simulink model "UUVModel"  (R2024b)
settings: Solver=ode4  StartTime=0.0  StopTime=100  FixedStep=0.001  RelTol=1e-3
PreLoadFcn:
  | [filepath,name,ext]  = fileparts(get_param(bdroot, 'FileName'));
  | InitFileName=[name,'_init.m'];
  | cd(filepath);
InitFcn:
  | [filepath,name,ext]  = fileparts(get_param(bdroot, 'FileName'));
  | InitFileName=[name,'_init.m'];
  | cd(filepath);
  | try
  | run(InitFileName);
  | end
values from neighbouring files (symbols this model uses):
  ESC = [ESC,ESCTmp]    [UUVModel_init.m]
  ModelParam_envAltitude = -600    [UUVModel_init.m]
  ModelParam_GPSLatLong = [ModelParam_envLatitude ModelParam_envLongitude]    [UUVModel_init.m]
  ModelParam_uavJ = [ModelParam_uavJxx,0,0;0,ModelParam_uavJyy,0;0,0,ModelParam_uavJzz]    [UUVModel_init.m]
  ModelParam_uavMass = 11.0    (= 11)    [UUVModel_init.m]
  ModelParam_uavType = int16(600)    [UUVModel_init.m]
  motor = [motor,motorTmp]    [UUVModel_init.m]
undefined symbols (not defined in the file or in its folder): Earth, ModelParam_timeSamp, UUV, WGS84
libraries: RflySimModelLab x15, aerolibtransform2 x2, aerolibatmos2 x2, sharedtransform x1, shared6dof x1, aerolibconvert2 x1, aerolibobsolete x1, aerolibasang x1, aerolibnav x1, aerolibgravity2 x1
(part 1 of 2)
settings Model: Creator=Jinrui  LastModifiedBy=12043
settings SolverCC: AlgebraicLoopSolver=TrustRegion
settings DataIOCC: ReturnWorkspaceOutputs=off
settings OptimizationCC: ReuseModelBlockBuffer=off  ZeroExternalMemoryAtStartup=off  ZeroInternalMemoryAtStartup=off  EfficientTunableParamExpr=on
settings DebuggingCC: ParameterTunabilityLossMsg=error  UnconnectedInputMsg=warning  UnconnectedOutputMsg=warning  UnconnectedLineMsg=warning  ArithmeticOperatorsInVariantConditions=warning
settings ModelReferenceCC: EnableRefExpFcnMdlSchedulingChecks=on
settings SFSimCC: SimUseLocalCustomCode=off  MATLABDynamicMemAlloc=off  CustomCodeUndefinedFunction=UseInterfaceOnly  SimTargetLang=C++
settings RTWCC: Description=Embedded Coder  SystemTargetFile=ert.tlc  GenerateMakefile=off  PackageGeneratedCodeAndArtifacts=on  PackageName=MulticopterModel  TemplateMakefile=ert_default_tmf  RTWUseLocalCustomCode=off  TargetLang=C++  RTWCompilerOptimization=on  GPUComputeCapability=3.5
settings CodeAppCC: ForceParamTrailComments=on  OperatorAnnotations=on  SimulinkDataObjDesc=on  SFDataObjDesc=on  MATLABFcnDesc=on  InsertBlockDesc=on  StateflowObjectComments=on  MATLABSourceComments=on
settings ERTTargetCC: TargetLangStandard=C++03 (ISO)  MultiwordLength=2048  GenerateSampleERTMain=on  CodeInterfacePackaging=C++ class  SupportContinuousTime=on  InlinedParameterPlacement=Hierarchical  MultiInstanceErrorCode=None  RootIOFormat=Structure reference  ERTCustomFileTemplate=example_file_process.tlc  ERTFilePackagingFormat=Compact  DynamicArrayContainerType=coder::array
settings SimscapeCC: SimscapeNormalizeSystem=off

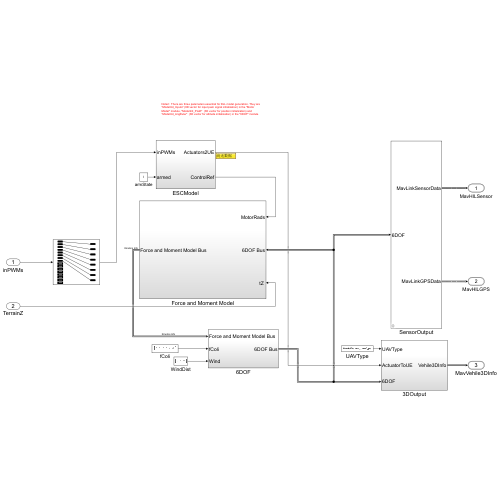
[thumbnail: Simulink's stored preview of the top-level diagram]
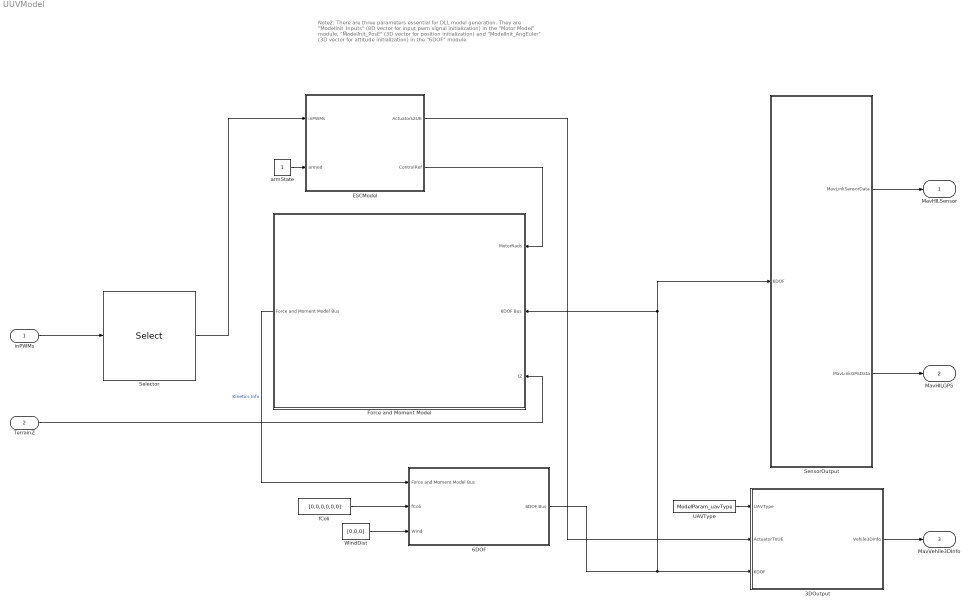
== system UUVModel ==
  note: Note2: There are three parameters essential for DLL model generation. They are "ModelInit_Inputs" (8D vector for input pwm signal initialization) in the "Motor Model" module, "ModelInit_PosE" (3D vector for position initialization) and "ModelInit_AngEuler" (3D vector for attitude initialization) in the "6DOF" module
  inPWMs : Inport  PortDimensions=16
  TerrainZ : Inport  Port=2
  3DOutput : Subsystem
  6DOF : Subsystem
  ESCModel : Subsystem
  Force and Moment Model : Subsystem
  Selector : Selector  InputPortWidth=16  IndexOptions=Index vector (dialog)  Indices=[1:8]  OutputSizes=1
  SensorOutput : Subsystem  mask{ModelParam_GPSLatLong=ModelParam_GPSLatLong, ModelParam_envAltitude=ModelParam_envAltitude}
      mask prompts: ModelParam_GPSLatLong "Initial latitude and longitude [deg]:"; ModelParam_envAltitude "Initial altitude [m]:"
      mask init:
      | ModelParam_GlobalNoiseGainSwitch =0.4;
      | %SimParam.timeACC=1;
      | %SimParam.timeStep=0.0001;
      | % SimParam.sonarSamp=0.1;
      | % SimParam.AngEularSamp=0.004;
      | % SimParam.AngRateSamp=0.004;
      | % SimParam.AccSensSamp=0.004;
      | % SimParam.GyroSensSamp=0.004;
      | % SimParam.AngQuaternSamp=0.004;
      | % SimParam.BaroSamp=0.008;
      | % SimParam.AngEulerSamp=0.004;
      | ModelParam_timeSampBaro = 0.01;
      | ModelParam_timeSampTurbWind = 0.01;
      | ModelParam_BusSampleRate = 0.001;
      | 
      | 
      | 
      | %%%ModelParam_BattModelEnable=int8(0);
      | %ModelParam_BattAuxCurrent=0.5;
      | %ModelParam_BattCells=3;
      | %ModelParam_BattCapacity=0.55;   %%这一项从模型配置界面传输给定
      | ModelParam_BattHoverMinutes=18;
      | ModelParam_BattHoverThr=0.609;
      | 
      | %GPS Parameter
      | ModelParam_GPSEphFinal=0.3;
      | ModelParam_GPSEpvFinal=0.4;
      | ModelParam_GPSFix3DFix=3;
      | ModelParam_GPSSatsVisible=10;
      | 
      | 
      | %Noise Parameter
      | ModelParam_noisePowerAccel = [0.001,0.001,0.003];%顺序 xyz 下同  不要修改这里
      | ModelParam_noiseSampleTimeAccel = 0.001;
      | %ModelParam_noiseLowPassFilterCoeAccel = 0.0001;
      | ModelParam_noisePowerOffGainAccel = 0.04;
      | ModelParam_noisePowerOffGainAccelZ = 0.03;
      | ModelParam_noisePowerOnGainAccel = 0.8;
      | ModelParam_noisePowerOnGainAccelZ = 4.5;
      | 
      | 
      | ModelParam_noisePowerGyro = [0.00001,0.00001,0.00001];%不要修改这里
      | ModelParam_noiseSampleTimeGyro = 0.001;
      | %ModelParam_noiseLowPassFilterCoeGyro = 0.0001;
      | ModelParam_noisePowerOffGainGyro = 0.02;
      | ModelParam_noisePowerOffGainGyroZ = 0.025;
      | ModelParam_noisePowerOnGainGyro = 2;%3.2;
      | ModelParam_noisePowerOnGainGyroZ = 1;
      | 
      | 
      | 
      | ModelParam_noisePowerMag = [0.00001,0.00001,0.00001];%不要修改这里
      | ModelParam_noiseSampleTimeMag = 0.01;
      | %ModelParam_noiseLowPassFilterCoeMag = 0.02;%暂时没有使用
      | ModelParam_noisePowerOffGainMag = 0.02;
      | ModelParam_noisePowerOffGainMagZ = 0.035;
      | ModelParam_noisePowerOnGainMag = 0.025;
      | ModelParam_noisePowerOnGainMagZ = 0.05;
      | 
      | 
      | 
      | ModelParam_noisePowerIMU=0;%IMU噪声，这里是白噪声，这里是经过归一化
      | 
      | ModelParam_noiseUpperGPS=0.5;  %GPS定位误差噪声，均匀噪声，这里填x,y,z的波动上限，单位是m
      | ModelParam_noiseGPSSampTime=0.02;%默认0.05
      | 
      | ModelParam_noiseUpperBaro=0; %气压计噪声，均匀噪声，这里填高度的波动上限，单位是m
      | ModelParam_noiseBaroSampTime=0.02;%气压计噪声更新频率，，默认0.05
      | ModelParam_noiseBaroCoupleWithSpeed=0;%气压计测量高度与动压关系，也就是风速与气压计掉高模型的系数，当前参数0.008飞机10m/s掉高1m
      | 
      | ModelParam_noiseUpperWindBodyRatio=0;%风波动系数，风速*(1+该系数)
      | ModelParam_noiseWindSampTime=0.001;
      | 
      | %%ModelParam_envGravityAcc = 9.81;
      | ModelParam_envAirDensity = 1.225;    %还没有用到
      | ModelParam_envDiffPressure = 0; % Differential pressure (airspeed) in millibar
      | ModelParam_noiseTs = 0.001;
      | 
      | %ModelParam_FailModelStartT = 5;
      | %ModelParam_FailModelLastT = 5;
  UAVType : Constant  Value=ModelParam_uavType
  WindDist : Constant  Value=[0,0,0]
  armState : Constant
  fColi : Constant  Value=[0,0,0,0,0,0]
  MavHILSensor : Outport  OutDataTypeStr=Bus: MavLinkSensor  VectorParamsAs1DForOutWhenUnconnected=off
  MavHILGPS : Outport  Port=2  OutDataTypeStr=Bus: MavLinkGPS  VectorParamsAs1DForOutWhenUnconnected=off
  MavVehile3DInfo : Outport  Port=3  OutDataTypeStr=Bus: MavVehileInfo  VectorParamsAs1DForOutWhenUnconnected=off
  wires:
  SensorOutput/1(MavLinkSensorData) -> MavHILSensor/1
  3DOutput/1(Vehile3DInfo) -> MavVehile3DInfo/1
  SensorOutput/2(MavLinkGPSData) -> MavHILGPS/1
  ESCModel/2(ControlRef) -> Force and Moment Model/1(MotorRads)
  Force and Moment Model/1(Force and Moment Model Bus) -> 6DOF/1(Force and Moment Model Bus)  "Kinetics Info"
  armState/1 -> ESCModel/2(armed)
  TerrainZ/1 -> Force and Moment Model/3("tZ ")
  inPWMs/1 -> Selector/1
  Selector/1 -> ESCModel/1(inPWMs)
  UAVType/1 -> 3DOutput/1(UAVType)
  6DOF/1(6DOF Bus) -> 3DOutput/3(6DOF), SensorOutput/1(6DOF), Force and Moment Model/2(6DOF Bus)
  ESCModel/1(Actuators2UE) -> 3DOutput/2(ActuatorToUE)
  WindDist/1 -> 6DOF/3(Wind)
  fColi/1 -> 6DOF/2(fColi)

== system UUVModel/3DOutput ==
  UAVType : Inport
  ActuatorToUE : Inport  Port=2
  6DOF : Inport  Port=3
  Bus Selector : BusSelector  OutputSignals=Ve,Xe,Eular(rad),DCM,wb,dwb/dt,AccB,WindB
  Clock1 : Clock
  Terminator : Terminator
  Terminator1 : Terminator
  Vehile3DModel : Subsystem
  Vehile3DInfo : Outport  VectorParamsAs1DForOutWhenUnconnected=off
  wires:
  Bus Selector/4 -> Vehile3DModel/9(<DCM>)  "<DCM>"
  Bus Selector/5 -> Vehile3DModel/6(<wb>)  "<wb>"
  Bus Selector/2 -> Vehile3DModel/7(<Xe>)  "<Xe>"
  UAVType/1 -> Vehile3DModel/1(vehicleType)
  ActuatorToUE/1 -> Vehile3DModel/2(ActuatorToUE)
  Vehile3DModel/1(Vehile3DInfo) -> Vehile3DInfo/1
  Clock1/1 -> Vehile3DModel/3(runnedTime)
  Bus Selector/3 -> Vehile3DModel/4(<Eular(rad)>)  "<Eular(rad)>"
  Bus Selector/1 -> Vehile3DModel/8(<Ve>)  "<Ve>"
  Bus Selector/7 -> Vehile3DModel/5(<AccB>)  "<AccB>"
  6DOF/1 -> Bus Selector/1
  Bus Selector/6 -> Terminator/1  "<dwb/dt>"
  Bus Selector/8 -> Terminator1/1  "<WindB>"

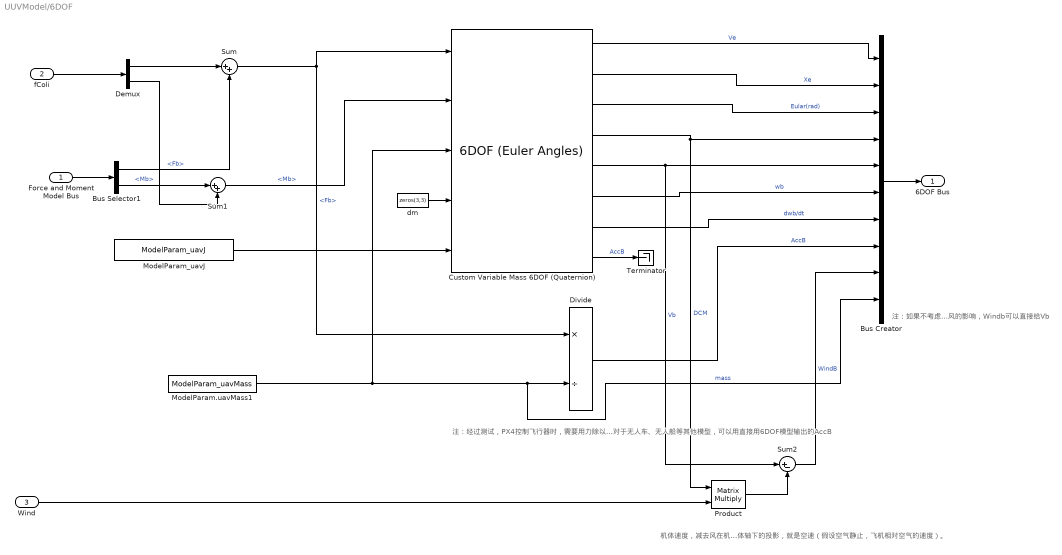
== system UUVModel/6DOF ==
  note: 注：如果不考虑风的影响，Windb可以直接给Vb
  note: 注：经过测试，PX4控制飞行器时，需要用力除以力矩的加速度去生成加速度计的数据，对于无人车、无人船等其他模型，可以用直接用6DOF模型输出的AccB
  note: 机体速度，减去风在机体轴下的投影，就是空速（假设空气静止，飞机相对空气的速度）。
  Force and Moment Model Bus : Inport
  fColi : Inport  Port=2
  Wind : Inport  Port=3
  Bus Creator : BusCreator  Inputs=10
  Bus Selector1 : BusSelector  OutputSignals=Fb,Mb
  Custom Variable Mass 6DOF (Quaternion) : shared6dof/6DOF (Euler Angles)  units=Metric (MKS)  mtype=Custom Variable  rep=Quaternion  xme_0=ModelInit_PosE  Vm_0=ModelInit_VelB  eul_0=ModelInit_AngEuler  pm_0=ModelInit_RateB  mass_0=ModelParam_uavMass  mass_e=0.5  mass_f=2.0  inertia=ModelParam_uavJ  inertia_e=eye(3)  inertia_f=2*eye(3)  k_quat=1.0  vre_flag=off  abi_flag=off  aMode=aMode  xme_statename=''  Vm_statename=''  eul_statename=''  quat_statename=''  pm_statename=''  mass_statename=''
  Demux : Demux  Outputs=2
  Divide : Product  Inputs=*/
  ModelParam.uavMass1 : Constant  Value=ModelParam_uavMass
  ModelParam_uavJ : Constant  Value=ModelParam_uavJ
  Product : Product  Multiplication=Matrix(*)
  Sum : Sum  Inputs=|++
  Sum1 : Sum  Inputs=|++
  Sum2 : Sum  Inputs=|+-
  Terminator : Terminator
  dm : Constant  Value=zeros(3,3)
  6DOF Bus : Outport  VectorParamsAs1DForOutWhenUnconnected=off
  wires:
  Bus Selector1/1 -> Sum/2  "<Fb>"
  Bus Selector1/2 -> Sum1/1  "<Mb>"
  Force and Moment Model Bus/1 -> Bus Selector1/1
  Demux/2 -> Sum1/2
  Demux/1 -> Sum/1
  fColi/1 -> Demux/1
  Custom Variable Mass 6DOF (Quaternion)/7 -> Bus Creator/7  "dwb/dt"
  Bus Creator/1 -> 6DOF Bus/1
  Custom Variable Mass 6DOF (Quaternion)/6 -> Bus Creator/6  "wb"
  Sum1/1 -> Custom Variable Mass 6DOF (Quaternion)/2  "<Mb>"
  Sum/1 -> Divide/1, Custom Variable Mass 6DOF (Quaternion)/1  "<Fb>"
  Custom Variable Mass 6DOF (Quaternion)/8 -> Terminator/1  "AccB"
  Custom Variable Mass 6DOF (Quaternion)/5 -> Sum2/1, Bus Creator/5  "Vb"
  Custom Variable Mass 6DOF (Quaternion)/4 -> Product/1, Bus Creator/4  "DCM"
  Custom Variable Mass 6DOF (Quaternion)/3 -> Bus Creator/3  "Eular(rad)"
  Custom Variable Mass 6DOF (Quaternion)/1 -> Bus Creator/1  "Ve"
  Custom Variable Mass 6DOF (Quaternion)/2 -> Bus Creator/2  "Xe"
  ModelParam.uavMass1/1 -> Bus Creator/10, Divide/2, Custom Variable Mass 6DOF (Quaternion)/3  "mass"
  Divide/1 -> Bus Creator/8  "AccB"
  Wind/1 -> Product/2
  Product/1 -> Sum2/2
  Sum2/1 -> Bus Creator/9  "WindB"
  dm/1 -> Custom Variable Mass 6DOF (Quaternion)/4
  ModelParam_uavJ/1 -> Custom Variable Mass 6DOF (Quaternion)/5

== system UUVModel/ESCModel ==
  note: 这个是输出给到UE用于舵机转动显示的，因此需要调整顺序到与UE对应，且修改单位到合适值。
  note: 输出的是8维向量
  inPWMs : Inport
  armed : Inport  Port=2
  ESC_All : Subsystem  AncestorBlock=RflySimModelLab/ESC_All  mask{ESCParam=ESC}
      mask prompts: ESCParam "电调参数"
      settings: LibrarySourceBlock=RflySimModelLab/ESC_All
  ToUEActuators : Subsystem
  Actuators2UE : Outport  VectorParamsAs1DForOutWhenUnconnected=off
  ControlRef : Outport  Port=2  VectorParamsAs1DForOutWhenUnconnected=off
  wires:
  inPWMs/1 -> ESC_All/1(inPWMs)
  ESC_All/1(MotorRads_reference) -> ToUEActuators/1(inMotorRads), ControlRef/1
  armed/1 -> ESC_All/2(armed)
  ToUEActuators/1(UERads) -> Actuators2UE/1

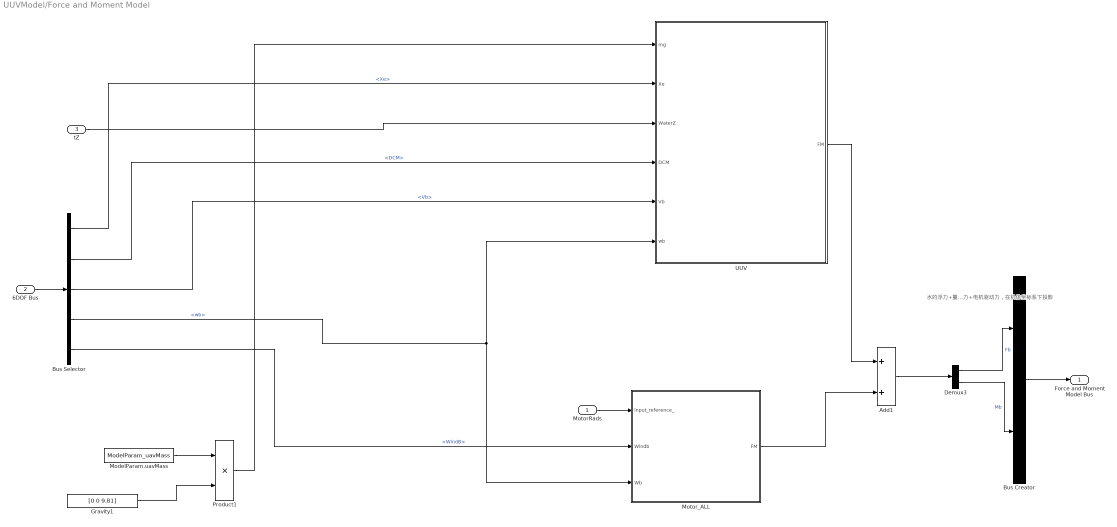
== system UUVModel/Force and Moment Model ==
  note: 水的浮力+重力+电机驱动力，在机体坐标系下投影
  MotorRads : Inport
  6DOF Bus : Inport  Port=2
  "tZ " : Inport  Port=3
  Add1 : Sum
  Bus Creator : BusCreator  Inputs=2
  Bus Selector : BusSelector  OutputSignals=Xe,DCM,Vb,wb,WindB
  Demux3 : Demux  Outputs=2
  Gravity1 : Constant  Value=[0 0 9.81]
  ModelParam.uavMass : Constant  Value=ModelParam_uavMass
  Motor_ALL : Subsystem  AncestorBlock=RflySimModelLab/Motor_ALL  mask{MotorParam=motor}
      mask prompts: MotorParam "电机参数"
      settings: LibrarySourceBlock=RflySimModelLab/Motor_ALL
  Product1 : Product
  UUV : Subsystem  AncestorBlock=RflySimModelLab/UUV  mask{ModelPara=UUV}
      mask prompts: ModelPara "水下无人机模型参数"
      settings: LibrarySourceBlock=RflySimModelLab/UUV
  Force and Moment Model Bus : Outport  VectorParamsAs1DForOutWhenUnconnected=off
  wires:
  Demux3/1 -> Bus Creator/1  "Fb"
  Gravity1/1 -> Product1/2
  ModelParam.uavMass/1 -> Product1/1
  Bus Creator/1 -> Force and Moment Model Bus/1
  6DOF Bus/1 -> Bus Selector/1
  Product1/1 -> UUV/1(mg)
  Demux3/2 -> Bus Creator/2  "Mb"
  Bus Selector/2 -> UUV/4(DCM)  "<DCM>"
  Motor_ALL/1(FM) -> Add1/2
  "tZ "/1 -> UUV/3(WaterZ)
  Bus Selector/1 -> UUV/2(Xe)  "<Xe>"
  Bus Selector/4 -> UUV/6(wb), Motor_ALL/3(Wb)  "<wb>"
  UUV/1(FM) -> Add1/1
  MotorRads/1 -> Motor_ALL/1(input_reference_)
  Add1/1 -> Demux3/1
  Bus Selector/3 -> UUV/5(Vb)  "<Vb>"
  Bus Selector/5 -> Motor_ALL/2(Windb)  "<WindB>"

== system UUVModel/SensorOutput ==
  note: Struct MavHILStateQuat{
      | uint64_t time_usec; /*< Timestamp (microseconds since UNIX epoch or microseconds since system boot)*/
      | float attitude_quaternion [ 4 ]; /*< Vehicle attitude expressed as normalized quaternion in w, x, y, z order (with 1 0 0 0 being the null-rotation)*/
      | float rollspeed; /*< Body frame roll / phi angular speed (rad/s)*/
      | float pitchspeed; /*< Body frame pitch / theta angular speed (rad/s)*/
      | float yawspeed; /*< Body frame yaw / psi angular speed (rad/s)*/
      | int32_t lat; /*< Latitude, expressed as * 1E7*/
      | int32_t lon; /*< Longitude, expressed as * 1E7*/
      | int32_t alt; /*< Altitude in meters, expressed as * 1000 (millimeters)*/
      | int16_t vx; /*< Ground X Speed (Latitude), expressed as cm/s*/
      | int16_t vy; /*< Ground Y Speed (Longitude), expressed as cm/s*/
      | int16_t vz; /*< Ground Z Speed (Altitude), expressed as cm/s*/
      | uint16_t ind_airspeed; /*< Indicated airspeed, expressed as cm/s*/
      | uint16_t true_airspeed; /*< True airspeed, expressed as cm/s*/
      | int16_t xacc; /*< X acceleration (mg)*/
      | int16_t yacc; /*< Y acceleration (mg)*/
      | int16_t zacc; /*< Z acceleration (mg)*/
      | };
  6DOF : Inport
  Bus Selector : BusSelector  OutputSignals=Ve,Xe,Eular(rad),DCM,wb,dwb/dt,AccB,WindB
  Bus Selector1 : BusSelector  OutputSignals=PosGPS,gravity,TempC,Rho
  Clock1 : Clock
  Data Type Conversion1 : DataTypeConversion  OutDataTypeStr=uint32  SaturateOnIntegerOverflow=off  RndMeth=Floor
  Environment Model : Subsystem
  Gain_clock : Gain  Gain=1E6
  HILGPSModel : Subsystem
  HILSensorMavModel : Subsystem
  Terminator : Terminator
  MavLinkSensorData : Outport  VectorParamsAs1DForOutWhenUnconnected=off
  MavLinkGPSData : Outport  Port=2  VectorParamsAs1DForOutWhenUnconnected=off
  wires:
  Bus Selector1/2 -> HILSensorMavModel/2(Gravity)  "<gravity>"
  Bus Selector/4 -> HILSensorMavModel/8(DCMbe)  "<DCM>"
  Bus Selector/6 -> HILSensorMavModel/6(dwt)  "<dwb/dt>"
  Bus Selector1/1 -> HILSensorMavModel/4(GPSPos)  "<PosGPS>"
  Bus Selector/7 -> HILSensorMavModel/7(Ab)  "<AccB>"
  Bus Selector/1 -> HILGPSModel/2(Ve)  "<Ve>"
  Bus Selector/5 -> HILSensorMavModel/5(wb)  "<wb>"
  Bus Selector/2 -> HILGPSModel/3(Xe)  "<Xe>"
  Bus Selector1/4 -> HILSensorMavModel/10(rho)  "<Rho>"
  Bus Selector1/3 -> HILSensorMavModel/3(TempC)  "<TempC>"
  Environment Model/1(Environment) -> Bus Selector1/1
  6DOF/1 -> Bus Selector/1, Environment Model/1(6DOF Bus)
  Clock1/1 -> Gain_clock/1
  Data Type Conversion1/1 -> HILGPSModel/1(time_usec), HILSensorMavModel/1(time_usec)  "time_usec"
  HILSensorMavModel/1(SensorOut) -> MavLinkSensorData/1
  Gain_clock/1 -> Data Type Conversion1/1
  HILGPSModel/1(MavLinkGPS) -> MavLinkGPSData/1
  Bus Selector/8 -> HILSensorMavModel/9(windB)  "<WindB>"
  Bus Selector/3 -> Terminator/1  "<Eular(rad)>"

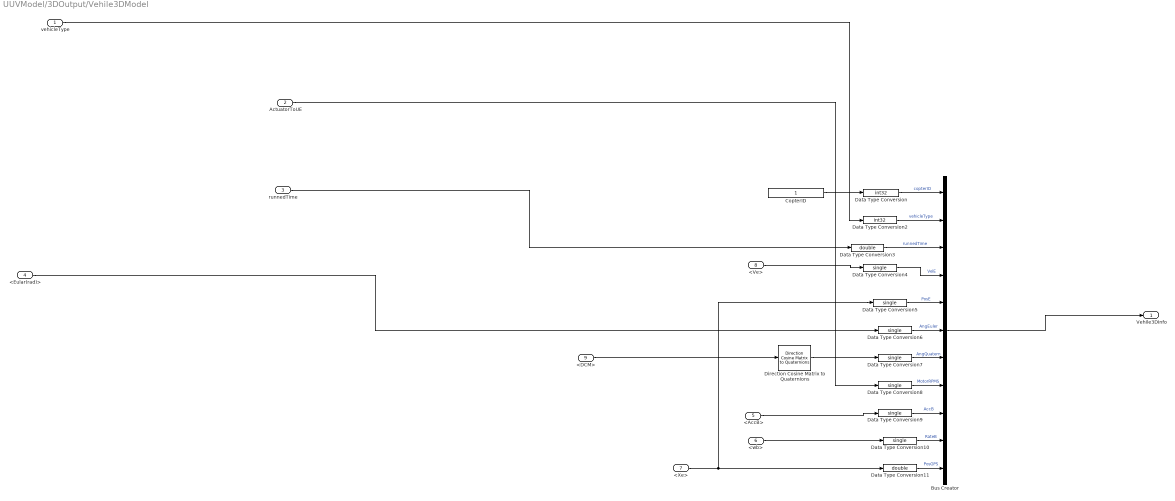
== system UUVModel/3DOutput/Vehile3DModel ==
  vehicleType : Inport
  ActuatorToUE : Inport  Port=2
  runnedTime : Inport  Port=3
  <Eular(rad)> : Inport  Port=4
  <AccB> : Inport  Port=5
  <wb> : Inport  Port=6
  <Xe> : Inport  Port=7
  <Ve> : Inport  Port=8
  <DCM> : Inport  Port=9
  Bus Creator : BusCreator  Inputs=11  OutDataTypeStr=Bus: MavVehileInfo
  CopterID : Constant
  Data Type Conversion : DataTypeConversion  OutDataTypeStr=int32  SaturateOnIntegerOverflow=off  RndMeth=Floor
  Data Type Conversion{4..10} (7 alike) : DataTypeConversion  OutDataTypeStr=single  SaturateOnIntegerOverflow=off  RndMeth=Floor
  Data Type Conversion11 : DataTypeConversion  OutDataTypeStr=double  SaturateOnIntegerOverflow=off  RndMeth=Floor
  Data Type Conversion2 : DataTypeConversion  OutDataTypeStr=int32  SaturateOnIntegerOverflow=off  RndMeth=Floor
  Data Type Conversion3 : DataTypeConversion  OutDataTypeStr=double  SaturateOnIntegerOverflow=off  RndMeth=Floor
  Direction Cosine Matrix to Quaternions : sharedtransform/Direction Cosine Matrix  to Quaternions  aMode=aMode  action=None  tolerance=eps(2)
  Vehile3DInfo : Outport  VectorParamsAs1DForOutWhenUnconnected=off
  wires:
  Bus Creator/1 -> Vehile3DInfo/1
  ActuatorToUE/1 -> Data Type Conversion8/1
  Data Type Conversion2/1 -> Bus Creator/2  "vehicleType"
  Data Type Conversion3/1 -> Bus Creator/3  "runnedTime"
  Data Type Conversion9/1 -> Bus Creator/9  "AccB"
  Data Type Conversion/1 -> Bus Creator/1  "copterID"
  Data Type Conversion7/1 -> Bus Creator/7  "AngQuatern"
  CopterID/1 -> Data Type Conversion/1
  Data Type Conversion10/1 -> Bus Creator/10  "RateB"
  Data Type Conversion6/1 -> Bus Creator/6  "AngEuler"
  Data Type Conversion5/1 -> Bus Creator/5  "PosE"
  Direction Cosine Matrix to Quaternions/1 -> Data Type Conversion7/1
  vehicleType/1 -> Data Type Conversion2/1
  Data Type Conversion4/1 -> Bus Creator/4  "VelE"
  Data Type Conversion8/1 -> Bus Creator/8  "MotorRPMS"
  Data Type Conversion11/1 -> Bus Creator/11  "PosGPS"
  <Eular(rad)>/1 -> Data Type Conversion6/1
  <Ve>/1 -> Data Type Conversion4/1
  <Xe>/1 -> Data Type Conversion5/1, Data Type Conversion11/1
  runnedTime/1 -> Data Type Conversion3/1
  <AccB>/1 -> Data Type Conversion9/1
  <wb>/1 -> Data Type Conversion10/1
  <DCM>/1 -> Direction Cosine Matrix to Quaternions/1

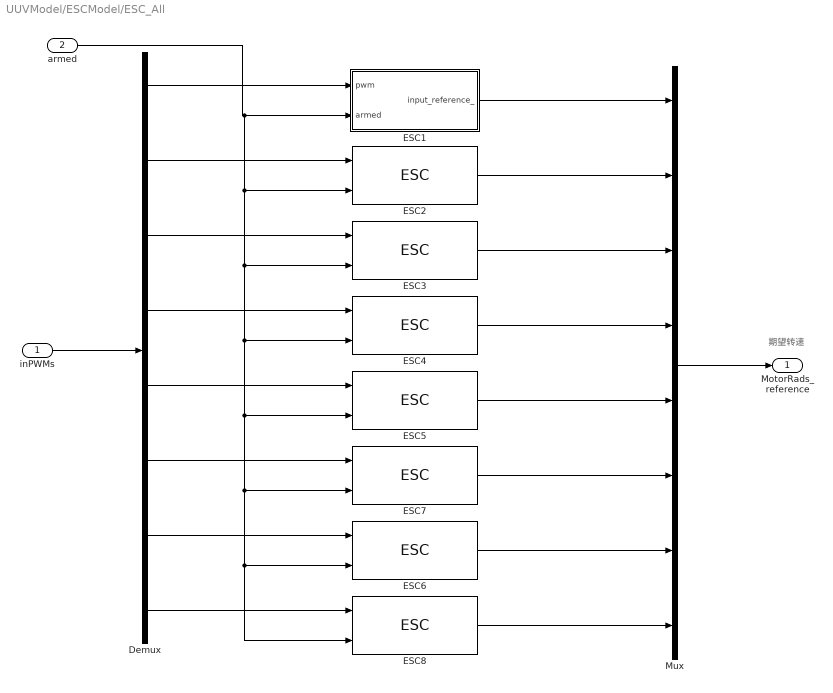
== system UUVModel/ESCModel/ESC_All ==
  note: 期望转速
  inPWMs : Inport  PortDimensions=8
  armed : Inport  Port=2  PortDimensions=1
  Demux : Demux  Outputs=8
  ESC1 : Subsystem  AncestorBlock=RflySimModelLab/ESC  mask{MotorPara=ESCParam(1)}
      mask prompts: MotorPara "电机名"
      settings: LibrarySourceBlock=RflySimModelLab/ESC
  ESC2 : RflySimModelLab/ESC  MotorPara=ESCParam(2)
  ESC3 : RflySimModelLab/ESC  MotorPara=ESCParam(3)
  ESC4 : RflySimModelLab/ESC  MotorPara=ESCParam(4)
  ESC5 : RflySimModelLab/ESC  MotorPara=ESCParam(5)
  ESC6 : RflySimModelLab/ESC  MotorPara=ESCParam(7)
  ESC7 : RflySimModelLab/ESC  MotorPara=ESCParam(6)
  ESC8 : RflySimModelLab/ESC  MotorPara=ESCParam(8)
  Mux : Mux  Inputs=8
  MotorRads_reference : Outport  VectorParamsAs1DForOutWhenUnconnected=off
  wires:
  armed/1 -> ESC1/2(armed), ESC2/2, ESC3/2, ESC4/2, ESC5/2, ESC7/2, ESC6/2, ESC8/2
  inPWMs/1 -> Demux/1
  Mux/1 -> MotorRads_reference/1
  ESC8/1 -> Mux/8
  Demux/8 -> ESC8/1
  ESC6/1 -> Mux/7
  Demux/7 -> ESC6/1
  ESC7/1 -> Mux/6
  Demux/6 -> ESC7/1
  ESC5/1 -> Mux/5
  Demux/5 -> ESC5/1
  ESC4/1 -> Mux/4
  Demux/4 -> ESC4/1
  ESC3/1 -> Mux/3
  Demux/3 -> ESC3/1
  Demux/1 -> ESC1/1(pwm)
  Demux/2 -> ESC2/1
  ESC1/1(input_reference_) -> Mux/1
  ESC2/1 -> Mux/2

== system UUVModel/ESCModel/ToUEActuators ==
  note: UE中水下无人艇的定义为
      | Rotor1：转每分
      | Rotor2：转每分
      | Rotor3：转每分
      | Rotor4：转每分
      | Rotor5：转每分
      | Rotor6：转每分
      | Rotor7：转每分
      | Rotor8：转每分
  note: inMotorRads取前8个元素的向量：
      |
      | Rotor1：转每分
      | Rotor2：转每分
      | Rotor3：转每分
      | Rotor4：转每分
      | Rotor5：转每分
      | Rotor6：转每分
      | Rotor7：转每分
      | Rotor8：转每分
  inMotorRads : Inport
  Demux : Demux  Outputs=8
  Gain : Gain  Gain=1/0.025
  Mux : Mux  Inputs=8
  UERads : Outport
  wires:
  inMotorRads/1 -> Demux/1
  Mux/1 -> Gain/1
  Demux/8 -> Mux/8
  Demux/1 -> Mux/1
  Demux/2 -> Mux/2
  Demux/3 -> Mux/3
  Demux/4 -> Mux/4
  Demux/5 -> Mux/5
  Demux/6 -> Mux/6
  Demux/7 -> Mux/7
  Gain/1 -> UERads/1

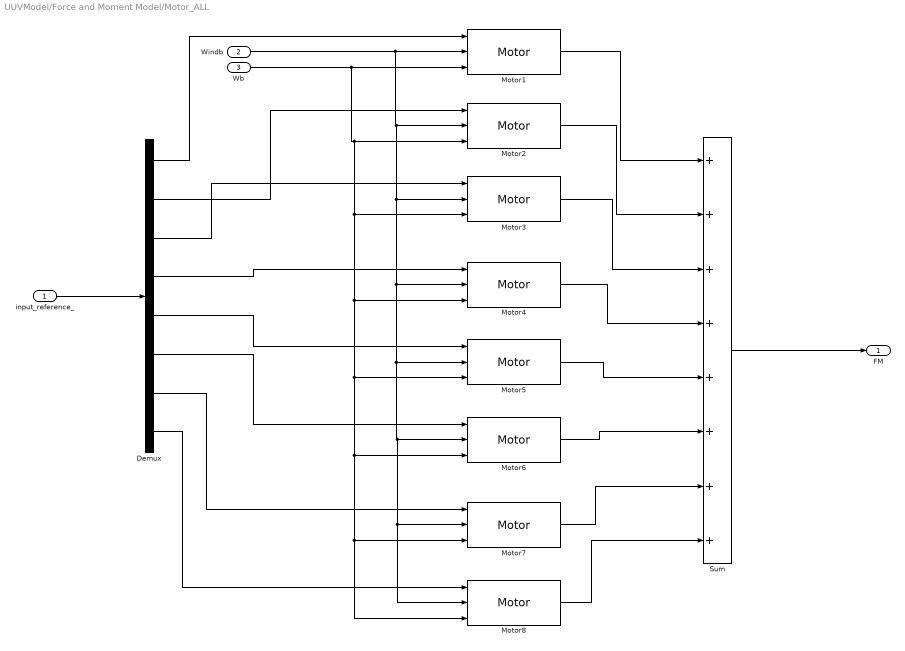
== system UUVModel/Force and Moment Model/Motor_ALL ==
  input_reference_ : Inport
  Windb : Inport  Port=2
  Wb : Inport  Port=3
  Demux : Demux  Outputs=8
  Motor1 : RflySimModelLab/Motor  MotorPara=MotorParam(1)
  Motor2 : RflySimModelLab/Motor  MotorPara=MotorParam(2)
  Motor3 : RflySimModelLab/Motor  MotorPara=MotorParam(3)
  Motor4 : RflySimModelLab/Motor  MotorPara=MotorParam(4)
  Motor5 : RflySimModelLab/Motor  MotorPara=MotorParam(5)
  Motor6 : RflySimModelLab/Motor  MotorPara=MotorParam(6)
  Motor7 : RflySimModelLab/Motor  MotorPara=MotorParam(7)
  Motor8 : RflySimModelLab/Motor  MotorPara=MotorParam(8)
  Sum : Sum  Inputs=++++++++
  FM : Outport
  wires:
  Demux/8 -> Motor8/1
  Demux/7 -> Motor7/1
  Demux/6 -> Motor6/1
  Demux/5 -> Motor5/1
  Demux/4 -> Motor4/1
  Demux/3 -> Motor3/1
  Demux/2 -> Motor2/1
  input_reference_/1 -> Demux/1
  Sum/1 -> FM/1
  Motor8/1 -> Sum/8
  Motor7/1 -> Sum/7
  Motor6/1 -> Sum/6
  Motor5/1 -> Sum/5
  Motor4/1 -> Sum/4
  Motor3/1 -> Sum/3
  Demux/1 -> Motor1/1
  Windb/1 -> Motor1/2, Motor2/2, Motor3/2, Motor4/2, Motor5/2, Motor6/2, Motor7/2, Motor8/2
  Wb/1 -> Motor1/3, Motor2/3, Motor3/3, Motor4/3, Motor6/3, Motor8/3, Motor7/3, Motor5/3
  Motor2/1 -> Sum/2
  Motor1/1 -> Sum/1

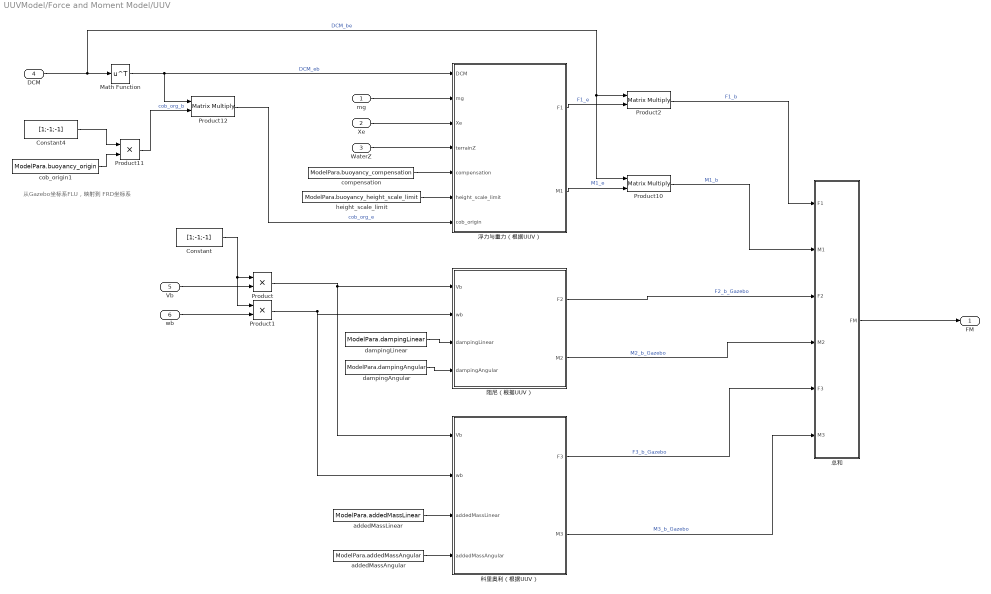
== system UUVModel/Force and Moment Model/UUV ==
  note: 从Gazebo坐标系FLU，映射到 FRD坐标系
  mg : Inport
  Xe : Inport  Port=2
  WaterZ : Inport  Port=3
  DCM : Inport  Port=4
  Vb : Inport  Port=5
  wb : Inport  Port=6
  Constant : Constant  Value=[1;-1;-1]
  Constant4 : Constant  Value=[1;-1;-1]
  Math Function : Math  Operator=transpose  SignedPower=on
  Product : Product
  Product1 : Product
  Product10 : Product  Multiplication=Matrix(*)
  Product11 : Product
  Product12 : Product  Multiplication=Matrix(*)
  Product2 : Product  Multiplication=Matrix(*)
  addedMassAngular : Constant  Value=ModelPara.addedMassAngular
  addedMassLinear : Constant  Value=ModelPara.addedMassLinear
  cob_origin1 : Constant  Value=ModelPara.buoyancy_origin
  compensation : Constant  Value=ModelPara.buoyancy_compensation
  dampingAngular : Constant  Value=ModelPara.dampingAngular
  dampingLinear : Constant  Value=ModelPara.dampingLinear
  height_scale_limit : Constant  Value=ModelPara.buoyancy_height_scale_limit
  总和 : Subsystem
  浮力与重力（根据UUV） : MATLAB Function  TreatAsAtomicUnit=on
  科里奥利（根据UUV） : MATLAB Function  TreatAsAtomicUnit=on
  阻尼（根据UUV） : MATLAB Function  TreatAsAtomicUnit=on
  FM : Outport
  wires:
  总和/1(FM) -> FM/1
  科里奥利（根据UUV）/2(M3) -> 总和/6(M3)  "M3_b_Gazebo"
  科里奥利（根据UUV）/1(F3) -> 总和/5(F3)  "F3_b_Gazebo"
  阻尼（根据UUV）/2(M2) -> 总和/4(M2)  "M2_b_Gazebo"
  阻尼（根据UUV）/1(F2) -> 总和/3(F2)  "F2_b_Gazebo"
  Product10/1 -> 总和/2(M1)  "M1_b"
  Product2/1 -> 总和/1(F1)  "F1_b"
  Math Function/1 -> Product12/1, 浮力与重力（根据UUV）/1(DCM)  "DCM_eb"
  DCM/1 -> Product2/1, Product10/1, Math Function/1  "DCM_be"
  Vb/1 -> Product/2
  Product12/1 -> 浮力与重力（根据UUV）/7(cob_origin)  "cob_org_e"
  Product11/1 -> Product12/2  "cob_org_b"
  Constant4/1 -> Product11/1
  cob_origin1/1 -> Product11/2
  浮力与重力（根据UUV）/2(M1) -> Product10/2  "M1_e"
  wb/1 -> Product1/2
  Product1/1 -> 阻尼（根据UUV）/2(wb), 科里奥利（根据UUV）/2(wb)
  Product/1 -> 阻尼（根据UUV）/1(Vb), 科里奥利（根据UUV）/1(Vb)
  Constant/1 -> Product/1, Product1/1
  WaterZ/1 -> 浮力与重力（根据UUV）/4(terrainZ)
  Xe/1 -> 浮力与重力（根据UUV）/3(Xe)
  mg/1 -> 浮力与重力（根据UUV）/2(mg)
  浮力与重力（根据UUV）/1(F1) -> Product2/2  "F1_e"
  addedMassLinear/1 -> 科里奥利（根据UUV）/3(addedMassLinear)
  addedMassAngular/1 -> 科里奥利（根据UUV）/4(addedMassAngular)
  dampingAngular/1 -> 阻尼（根据UUV）/4(dampingAngular)
  dampingLinear/1 -> 阻尼（根据UUV）/3(dampingLinear)
  height_scale_limit/1 -> 浮力与重力（根据UUV）/6(height_scale_limit)
  compensation/1 -> 浮力与重力（根据UUV）/5(compensation)

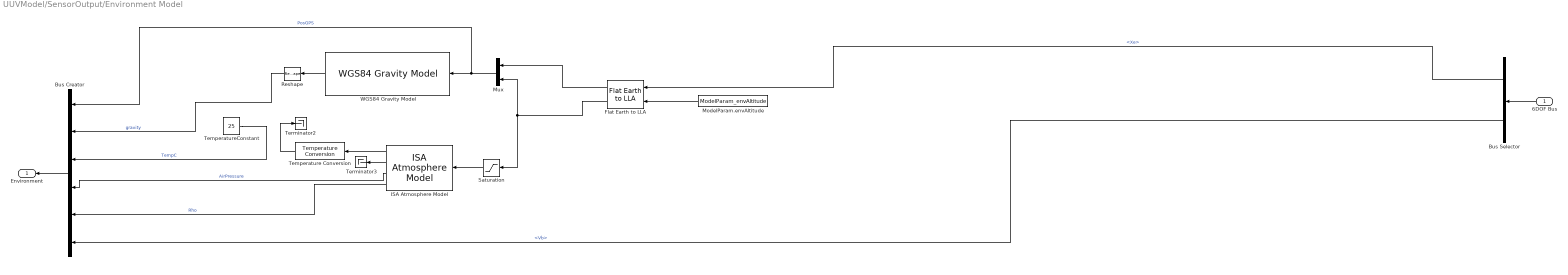
== system UUVModel/SensorOutput/Environment Model ==
  6DOF Bus : Inport
  Bus Creator : BusCreator  Inputs=6
  Bus Selector : BusSelector  OutputSignals=Xe,Vb
  Flat Earth to LLA : aerolibtransform2/Flat Earth to LLA  units=Metric (MKS)  ptype=Earth (WGS84)  F=1/298.257223563  R=6378137  refPosPort=off  LL0=ModelParam_GPSLatLong  psi=0
  ISA Atmosphere Model : aerolibatmos2/ISA Atmosphere Model  useExtended=off  action=Warning  custom=off  viscosityOut=off  g=9.80665  gamma=1.4  R=287.0531  L=0.0065  h_trop=11000  h_strat=20000  rho0=1.225  P0=101325  T0=288.15  h0=0  S=110.4  Tref=273.15  muref=1.716e-5
  ModelParam.envAltitude : Constant  Value=ModelParam_envAltitude
  Mux : Mux  Inputs=2
  Reshape : Reshape
  Saturation : Saturate  UpperLimit=100000  LowerLimit=0
  Temperature Conversion : aerolibconvert2/Temperature Conversion  IU=K  OU=C
  TemperatureConstant : Constant  Value=25
  Terminator2 : Terminator
  Terminator3 : Terminator
  "WGS84 Gravity Model " : aerolibobsolete/WGS84 Gravity Model   model=WGS84 Taylor Series  units=Metric (MKS)  no_atmos=on  precessing=on  jd_loc=off  month=October  day=10  year=2004  no_centrifugal=on  action=Warning
  Environment : Outport  VectorParamsAs1DForOutWhenUnconnected=off
  wires:
  "WGS84 Gravity Model "/1 -> Reshape/1
  Reshape/1 -> Bus Creator/2  "gravity"
  ISA Atmosphere Model/1 -> Temperature Conversion/1
  ISA Atmosphere Model/2 -> Terminator3/1
  ISA Atmosphere Model/3 -> Bus Creator/4  "AirPressure"
  ISA Atmosphere Model/4 -> Bus Creator/5  "Rho"
  Mux/1 -> Bus Creator/1, "WGS84 Gravity Model "/1  "PosGPS"
  Flat Earth to LLA/1 -> Mux/1
  Bus Selector/2 -> Bus Creator/6  "<Vb>"
  Temperature Conversion/1 -> Terminator2/1
  TemperatureConstant/1 -> Bus Creator/3  "TempC"
  6DOF Bus/1 -> Bus Selector/1
  Bus Selector/1 -> Flat Earth to LLA/1  "<Xe>"
  Bus Creator/1 -> Environment/1
  Flat Earth to LLA/2 -> Mux/2, Saturation/1
  Saturation/1 -> ISA Atmosphere Model/1
  ModelParam.envAltitude/1 -> Flat Earth to LLA/2

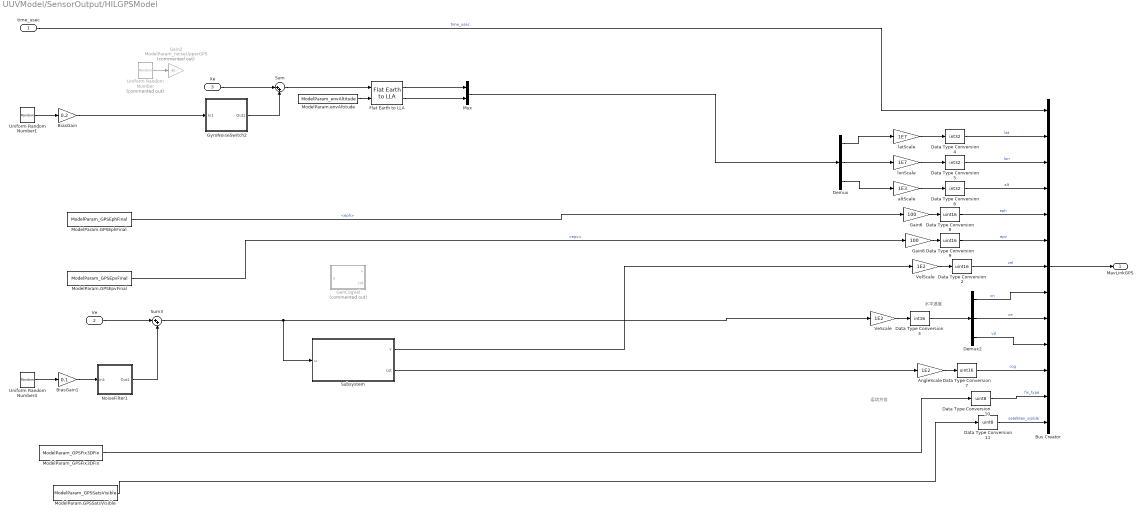
== system UUVModel/SensorOutput/HILGPSModel ==
  note: 水平速度
  note: 运动方位
  time_usec : Inport
  Ve : Inport  Port=2
  Xe : Inport  Port=3
  AngleScale : Gain  Gain=1E2
  BiasGain : Gain  Gain=0.2
  BiasGain1 : Gain  Gain=0.1
  Bus Creator : BusCreator  Inputs=13  OutDataTypeStr=Bus: MavLinkGPS  NonVirtualBus=on
  Data Type Conversion10 : DataTypeConversion  OutDataTypeStr=uint8  RndMeth=Round  SaturateOnIntegerOverflow=off
  Data Type Conversion11 : DataTypeConversion  OutDataTypeStr=uint8  RndMeth=Round  SaturateOnIntegerOverflow=off
  Data Type Conversion{2,7..9} (4 alike) : DataTypeConversion  OutDataTypeStr=uint16  RndMeth=Round  SaturateOnIntegerOverflow=off
  Data Type Conversion3 : DataTypeConversion  OutDataTypeStr=int16  RndMeth=Round  SaturateOnIntegerOverflow=off
  Data Type Conversion4 : DataTypeConversion  OutDataTypeStr=int32  RndMeth=Round  SaturateOnIntegerOverflow=off
  Data Type Conversion5 : DataTypeConversion  OutDataTypeStr=int32  RndMeth=Round  SaturateOnIntegerOverflow=off
  Data Type Conversion6 : DataTypeConversion  OutDataTypeStr=int32  RndMeth=Round  SaturateOnIntegerOverflow=off
  Demux : Demux  Outputs=3
  Demux2 : Demux  Outputs=3
  Flat Earth to LLA : aerolibtransform2/Flat Earth to LLA  units=Metric (MKS)  ptype=Earth (WGS84)  F=1/298.257223563  R=6378137  refPosPort=off  LL0=ModelParam_GPSLatLong  psi=0
  Gain2 : Gain  Commented=on  Gain=ModelParam_noiseUpperGPS
  Gain6 : Gain  Gain=100
  Gain8 : Gain  Gain=100
  GenCogVel : MATLAB Function  Commented=on  TreatAsAtomicUnit=on
  GyroNoiseSwitch2 : Subsystem
  ModelParam.GPSEphFinal : Constant  Value=ModelParam_GPSEphFinal
  ModelParam.GPSEpvFinal : Constant  Value=ModelParam_GPSEpvFinal
  ModelParam.GPSSatsVisible : Constant  Value=ModelParam_GPSSatsVisible
  ModelParam.envAltitude : Constant  Value=ModelParam_envAltitude
  ModelParam_GPSFix3DFix : Constant  Value=ModelParam_GPSFix3DFix
  Mux : Mux  Inputs=2
  NoiseFilter1 : Subsystem
  Subsystem : Subsystem
  Sum : Sum  Inputs=|++
  Sum3 : Sum  Inputs=|++
  Uniform Random Number : UniformRandomNumber  Commented=on  Minimum=[-1,-1,-3]  Maximum=[1,1,3]  Seed=[14524,7875,698]  SampleTime=ModelParam_timeSamp
  Uniform Random Number1 : UniformRandomNumber  Minimum=[-1,-1,-2]  Maximum=[1,1,2]  Seed=[1452,787,69]  SampleTime=0.02
  Uniform Random Number4 : UniformRandomNumber  Minimum=[-1,-1,-2]  Maximum=[1,1,2]  Seed=[5445,45433,33433]  SampleTime=0.02
  VeScale : Gain  Gain=1E2
  VelScale : Gain  Gain=1E2
  altScale : Gain  Gain=1E3
  latScale : Gain  Gain=1E7
  lonScale : Gain  Gain=1E7
  MavLinkGPS : Outport  VectorParamsAs1DForOutWhenUnconnected=off
  wires:
  Data Type Conversion8/1 -> Bus Creator/5  "eph"
  Gain8/1 -> Data Type Conversion9/1
  Gain6/1 -> Data Type Conversion8/1
  Data Type Conversion9/1 -> Bus Creator/6  "epv"
  time_usec/1 -> Bus Creator/1  "time_usec"
  latScale/1 -> Data Type Conversion4/1
  lonScale/1 -> Data Type Conversion5/1
  altScale/1 -> Data Type Conversion6/1
  Data Type Conversion4/1 -> Bus Creator/2  "lat"
  Data Type Conversion5/1 -> Bus Creator/3  "lon"
  Data Type Conversion6/1 -> Bus Creator/4  "alt"
  Demux2/1 -> Bus Creator/8  "vn"
  Demux2/2 -> Bus Creator/9  "ve"
  Demux2/3 -> Bus Creator/10  "vd"
  VeScale/1 -> Data Type Conversion3/1
  Data Type Conversion3/1 -> Demux2/1
  VelScale/1 -> Data Type Conversion2/1
  Data Type Conversion2/1 -> Bus Creator/7  "vel"
  AngleScale/1 -> Data Type Conversion7/1
  Data Type Conversion7/1 -> Bus Creator/11  "cog"
  ModelParam.GPSSatsVisible/1 -> Data Type Conversion11/1
  Flat Earth to LLA/2 -> Mux/2
  ModelParam.envAltitude/1 -> Flat Earth to LLA/2
  Xe/1 -> Sum/1
  Flat Earth to LLA/1 -> Mux/1
  Uniform Random Number/1 -> Gain2/1
  Sum/1 -> Flat Earth to LLA/1
  Uniform Random Number1/1 -> BiasGain/1
  BiasGain/1 -> GyroNoiseSwitch2/1(In1)
  Mux/1 -> Demux/1
  ModelParam_GPSFix3DFix/1 -> Data Type Conversion10/1
  Ve/1 -> Sum3/1
  GyroNoiseSwitch2/1(Out1) -> Sum/2
  Bus Creator/1 -> MavLinkGPS/1
  BiasGain1/1 -> NoiseFilter1/1(In1)
  Uniform Random Number4/1 -> BiasGain1/1
  Sum3/1 -> Subsystem/1(u), VeScale/1
  NoiseFilter1/1(Out1) -> Sum3/2
  Demux/2 -> lonScale/1
  ModelParam.GPSEpvFinal/1 -> Gain8/1  "<epv>"
  Demux/3 -> altScale/1
  ModelParam.GPSEphFinal/1 -> Gain6/1  "<eph>"
  Subsystem/1(v) -> VelScale/1
  Subsystem/2(cot) -> AngleScale/1
  Data Type Conversion11/1 -> Bus Creator/13  "satellites_visible"
  Data Type Conversion10/1 -> Bus Creator/12  "fix_type"
  Demux/1 -> latScale/1

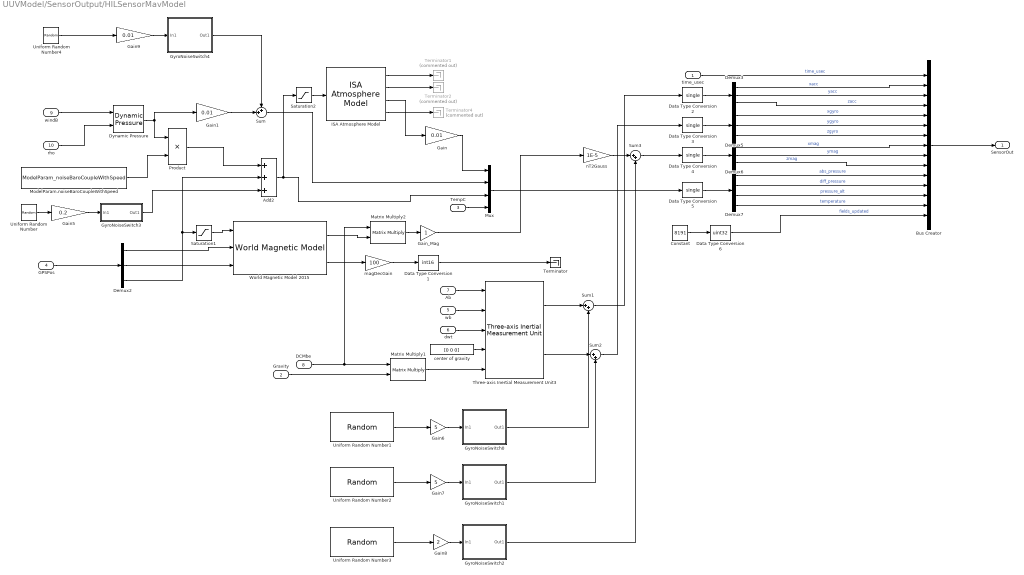
== system UUVModel/SensorOutput/HILSensorMavModel ==
  time_usec : Inport
  Gravity : Inport  Port=2
  TempC : Inport  Port=3
  GPSPos : Inport  Port=4
  wb : Inport  Port=5
  dwt : Inport  Port=6
  Ab : Inport  Port=7
  DCMbe : Inport  Port=8
  windB : Inport  Port=9
  rho : Inport  Port=10
  Add2 : Sum  Inputs=+++
  Bus Creator : BusCreator  Inputs=15  OutDataTypeStr=Bus: MavLinkSensor  NonVirtualBus=on
  Constant : Constant  Value=8191
  Data Type Conversion1 : DataTypeConversion  OutDataTypeStr=int16  SaturateOnIntegerOverflow=off  RndMeth=Floor
  Data Type Conversion{2..5} (4 alike) : DataTypeConversion  OutDataTypeStr=single  SaturateOnIntegerOverflow=off  RndMeth=Floor
  Data Type Conversion6 : DataTypeConversion  OutDataTypeStr=uint32  SaturateOnIntegerOverflow=off  RndMeth=Floor
  Demux{2..3,5..6} (4 alike) : Demux  Outputs=3
  Demux7 : Demux
  Dynamic Pressure : aerolibasang/Dynamic Pressure
  Gain : Gain  Gain=0.01
  Gain1 : Gain  Gain=0.01
  Gain5 : Gain  Gain=0.2
  Gain6 : Gain  Gain=5
  Gain7 : Gain  Gain=5
  Gain8 : Gain  Gain=2
  Gain9 : Gain  Gain=0.01
  Gain_Mag : Gain
  GyroNoiseSwitch0 : Subsystem
  GyroNoiseSwitch1 : Subsystem
  GyroNoiseSwitch2 : Subsystem
  GyroNoiseSwitch3 : Subsystem
  GyroNoiseSwitch4 : Subsystem
  ISA Atmosphere Model : aerolibatmos2/ISA Atmosphere Model  useExtended=off  action=Warning  custom=off  viscosityOut=off  g=9.80665  gamma=1.4  R=287.0531  L=0.0065  h_trop=11000  h_strat=20000  rho0=1.225  P0=101325  T0=288.15  h0=0  S=110.4  Tref=273.15  muref=1.716e-5
  Matrix Multiply1 : Product  Multiplication=Matrix(*)
  Matrix Multiply2 : Product  Multiplication=Matrix(*)
  ModelParam.noiseBaroCoupleWithSpeed : Constant  Value=ModelParam_noiseBaroCoupleWithSpeed
  Mux : Mux
  Product : Product
  Saturation1 : Saturate  UpperLimit=100000  LowerLimit=0
  Saturation2 : Saturate  UpperLimit=100000  LowerLimit=0
  Sum : Sum  Inputs=++|
  Sum1 : Sum  Inputs=|++
  Sum2 : Sum  Inputs=|++
  Sum3 : Sum  Inputs=|++
  Terminator : Terminator
  Terminator1 : Terminator  Commented=on
  Terminator2 : Terminator  Commented=on
  Terminator4 : Terminator  Commented=on
  Three-axis Inertial Measurement Unit3 : aerolibnav/Three-axis Inertial Measurement Unit  units=Metric (MKS)  imu=[0 0 0]  i_Ts=0  dtype_a=on  w_a=190  z_a=0.707  a_sf_cc=[1 0 0; 0 1 0; 0 0 1]  a_bias=[0 0 0]  a_sat="[-160  -160  -160 160 160 160]"  dtype_g=on  w_g=190  z_g=0.707  g_sf_cc=[1 0 0; 0 1 0; 0 0 1]  g_bias=[0 0 0]  g_sens=[0 0 0]  g_sat="[-4.36  -4.36  -4.36 4.36 4.36 4.36]"  i_rand=off  i_seeds=[23093 23094 23095 23096 23097 23098]  i_pow=ModelParam_noisePowerIMU*[0.0000005 0.0000005 0.0000005 0.000000002 0.000000002 0.000000002]
  Uniform Random Number : UniformRandomNumber  Minimum=-2  Maximum=2  Seed=15634  SampleTime=0.01
  Uniform Random Number1 : UniformRandomNumber  Minimum=-[0.1,0.1,0.2]  Maximum=[0.1,0.1,0.2]  Seed=[12233,645554,678766]  SampleTime=0.004
  Uniform Random Number2 : UniformRandomNumber  Minimum=-[0.01,0.01,0.01]  Maximum=[0.01,0.01,0.01]  Seed=[3243,44556,2334343]  SampleTime=0.004
  Uniform Random Number3 : UniformRandomNumber  Minimum=-[0.01,0.01,0.01]  Maximum=[0.01,0.01,0.01]  Seed=[45465,454534,1234232]  SampleTime=0.004
  Uniform Random Number4 : UniformRandomNumber  Seed=25634  SampleTime=0.01
  World Magnetic Model 2015 : aerolibgravity2/World Magnetic Model  model=WMM2015 V2 (2015-2020)  customFile='WMM2020.COF'  units=Metric (MKS)  time_in=off  month=November  day=3  year=2017  action=Error  h_out=off  dec_out=on  inc_out=off  ti_out=off
  center of gravity : Constant  Value=[0 0 0]
  magDecGain : Gain  Gain=100
  nT2Gauss : Gain  Gain=1E-5
  SensorOut : Outport  VectorParamsAs1DForOutWhenUnconnected=off
  wires:
  center of gravity/1 -> Three-axis Inertial Measurement Unit3/4
  Sum1/1 -> Data Type Conversion2/1
  Sum2/1 -> Data Type Conversion3/1
  Sum3/1 -> Data Type Conversion4/1
  Matrix Multiply2/1 -> Gain_Mag/1
  magDecGain/1 -> Data Type Conversion1/1
  GyroNoiseSwitch3/1(Out1) -> Add2/3
  Product/1 -> Add2/1
  ModelParam.noiseBaroCoupleWithSpeed/1 -> Product/2
  rho/1 -> Dynamic Pressure/2
  windB/1 -> Dynamic Pressure/1
  Uniform Random Number/1 -> Gain5/1
  dwt/1 -> Three-axis Inertial Measurement Unit3/3
  Gain_Mag/1 -> nT2Gauss/1
  Dynamic Pressure/1 -> Gain1/1, Product/1
  Add2/1 -> Mux/3, Saturation2/1
  Demux2/3 -> Saturation1/1, Add2/2
  Demux2/2 -> World Magnetic Model 2015/3
  Demux2/1 -> World Magnetic Model 2015/2
  Matrix Multiply1/1 -> Three-axis Inertial Measurement Unit3/5
  DCMbe/1 -> Matrix Multiply2/1, Matrix Multiply1/1
  Gravity/1 -> Matrix Multiply1/2
  Sum/1 -> Mux/2
  Gain/1 -> Mux/1
  Data Type Conversion6/1 -> Bus Creator/15  "fields_updated"
  Constant/1 -> Data Type Conversion6/1
  time_usec/1 -> Bus Creator/1  "time_usec"
  Demux7/2 -> Bus Creator/12  "diff_pressure"
  Demux7/3 -> Bus Creator/13  "pressure_alt"
  Demux6/2 -> Bus Creator/9  "ymag"
  Demux6/3 -> Bus Creator/10  "zmag"
  TempC/1 -> Mux/4
  Mux/1 -> Data Type Conversion5/1
  Demux7/1 -> Bus Creator/11  "abs_pressure"
  Demux5/2 -> Bus Creator/6  "ygyro"
  Demux6/1 -> Bus Creator/8  "xmag"
  Demux5/3 -> Bus Creator/7  "zgyro"
  Demux7/4 -> Bus Creator/14  "temperature"
  Demux3/1 -> Bus Creator/2  "xacc"
  Demux3/2 -> Bus Creator/3  "yacc"
  Demux5/1 -> Bus Creator/5  "xgyro"
  Demux3/3 -> Bus Creator/4  "zacc"
  Ab/1 -> Three-axis Inertial Measurement Unit3/1
  wb/1 -> Three-axis Inertial Measurement Unit3/2
  nT2Gauss/1 -> Sum3/1
  Gain8/1 -> GyroNoiseSwitch2/1(In1)
  GyroNoiseSwitch1/1(Out1) -> Sum2/2
  GyroNoiseSwitch2/1(Out1) -> Sum3/2
  Data Type Conversion2/1 -> Demux3/1
  Data Type Conversion3/1 -> Demux5/1
  Data Type Conversion4/1 -> Demux6/1
  Data Type Conversion5/1 -> Demux7/1
  Bus Creator/1 -> SensorOut/1
  Data Type Conversion1/1 -> Terminator/1
  Three-axis Inertial Measurement Unit3/1 -> Sum1/1
  Three-axis Inertial Measurement Unit3/2 -> Sum2/1
  ISA Atmosphere Model/2 -> Terminator2/1
  ISA Atmosphere Model/4 -> Terminator4/1
  ISA Atmosphere Model/1 -> Terminator1/1
  Gain5/1 -> GyroNoiseSwitch3/1(In1)
  GyroNoiseSwitch0/1(Out1) -> Sum1/2
  Uniform Random Number1/1 -> Gain6/1
  Gain7/1 -> GyroNoiseSwitch1/1(In1)
  Uniform Random Number2/1 -> Gain7/1
  Uniform Random Number3/1 -> Gain8/1
  ISA Atmosphere Model/3 -> Gain/1
  Gain6/1 -> GyroNoiseSwitch0/1(In1)
  Gain9/1 -> GyroNoiseSwitch4/1(In1)
  Uniform Random Number4/1 -> Gain9/1
  Gain1/1 -> Sum/2
  GyroNoiseSwitch4/1(Out1) -> Sum/1
  Saturation1/1 -> World Magnetic Model 2015/1
  Saturation2/1 -> ISA Atmosphere Model/1
  World Magnetic Model 2015/2 -> magDecGain/1
  World Magnetic Model 2015/1 -> Matrix Multiply2/2
  GPSPos/1 -> Demux2/1

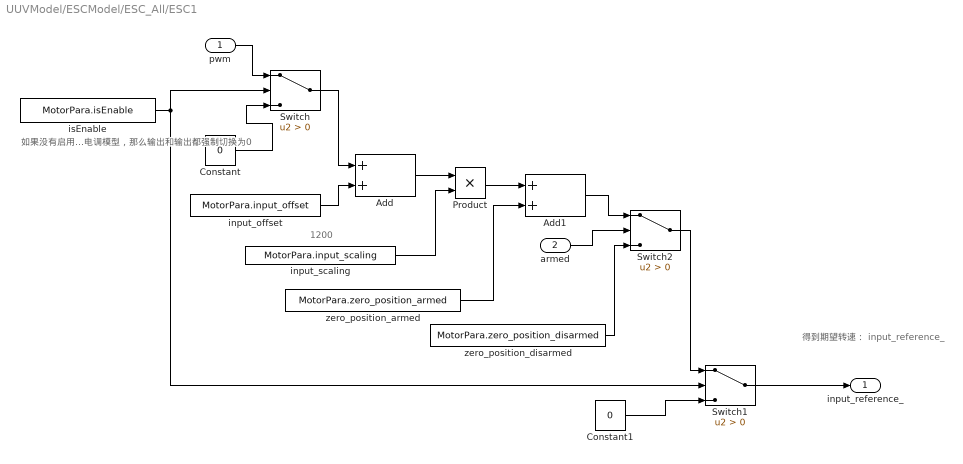
== system UUVModel/ESCModel/ESC_All/ESC1 ==
  note: 得到期望转速：
      | input_reference_
  note: 1200
  note: 如果没有启用电调模型，那么输出和输出都强制切换为0
  pwm : Inport
  armed : Inport  Port=2
  Add : Sum
  Add1 : Sum
  Constant : Constant  Value=0
  Constant1 : Constant  Value=0
  Product : Product
  Switch : Switch  Criteria=u2 > Threshold  SaturateOnIntegerOverflow=off  InputSameDT=off
  Switch1 : Switch  Criteria=u2 > Threshold  SaturateOnIntegerOverflow=off  InputSameDT=off
  Switch2 : Switch  Criteria=u2 > Threshold  SaturateOnIntegerOverflow=off  InputSameDT=off
  input_offset : Constant  Value=MotorPara.input_offset
  input_scaling : Constant  Value=MotorPara.input_scaling
  isEnable : Constant  Value=MotorPara.isEnable
  zero_position_armed : Constant  Value=MotorPara.zero_position_armed
  zero_position_disarmed : Constant  Value=MotorPara.zero_position_disarmed
  input_reference_ : Outport  VectorParamsAs1DForOutWhenUnconnected=off
  wires:
  zero_position_disarmed/1 -> Switch2/3
  Add1/1 -> Switch2/1
  armed/1 -> Switch2/2
  Constant1/1 -> Switch1/3
  Switch/1 -> Add/1
  Constant/1 -> Switch/3
  isEnable/1 -> Switch/2, Switch1/2
  Add/1 -> Product/1
  input_offset/1 -> Add/2
  Switch2/1 -> Switch1/1
  pwm/1 -> Switch/1
  input_scaling/1 -> Product/2
  Product/1 -> Add1/1
  zero_position_armed/1 -> Add1/2
  Switch1/1 -> input_reference_/1

== system UUVModel/Force and Moment Model/UUV/总和 ==
  F1 : Inport
  M1 : Inport  Port=2
  F2 : Inport  Port=3
  M2 : Inport  Port=4
  F3 : Inport  Port=5
  M3 : Inport  Port=6
  Add1 : Sum  Inputs=+++
  Add2 : Sum  Inputs=+++
  Constant2 : Constant  Value=[1;-1;-1]
  Mux : Mux  Inputs=2
  Product5 : Product
  Product6 : Product
  FM : Outport  VectorParamsAs1DForOutWhenUnconnected=off
  wires:
  M3/1 -> Add2/3
  M2/1 -> Add2/2
  Add2/1 -> Product6/2
  Mux/1 -> FM/1
  Constant2/1 -> Product5/1, Product6/1
  Product5/1 -> Mux/1  "F"
  Add1/1 -> Product5/2
  F1/1 -> Add1/1
  M1/1 -> Add2/1
  F3/1 -> Add1/3
  Product6/1 -> Mux/2  "M"
  F2/1 -> Add1/2

== system UUVModel/SensorOutput/HILGPSModel/GyroNoiseSwitch2 ==
  In1 : Inport
  Constant1 : Constant  Value=ModelParam_GlobalNoiseGainSwitch
  Constant2 : Constant  Value=0.3
  Gain2 : Gain  Gain=0.7
  Product4 : Product
  Sum : Sum  Inputs=|++
  Out1 : Outport  VectorParamsAs1DForOutWhenUnconnected=off
  wires:
  Sum/1 -> Product4/2
  Product4/1 -> Out1/1
  Gain2/1 -> Sum/1
  In1/1 -> Product4/1
  Constant1/1 -> Gain2/1
  Constant2/1 -> Sum/2

== system UUVModel/SensorOutput/HILGPSModel/NoiseFilter1 ==
  In1 : Inport
  Demux : Demux  Outputs=3
  Mux1 : Mux  Inputs=3
  Transfer Fcn1 : TransferFcn  Denominator=[0.05 1]
  Transfer Fcn2 : TransferFcn  Denominator=[0.05 1]
  Transfer Fcn4 : TransferFcn  Denominator=[0.05 1]
  Out1 : Outport  VectorParamsAs1DForOutWhenUnconnected=off
  wires:
  Mux1/1 -> Out1/1
  In1/1 -> Demux/1
  Demux/3 -> Transfer Fcn2/1
  Transfer Fcn4/1 -> Mux1/1
  Transfer Fcn2/1 -> Mux1/3
  Demux/1 -> Transfer Fcn4/1
  Transfer Fcn1/1 -> Mux1/2
  Demux/2 -> Transfer Fcn1/1

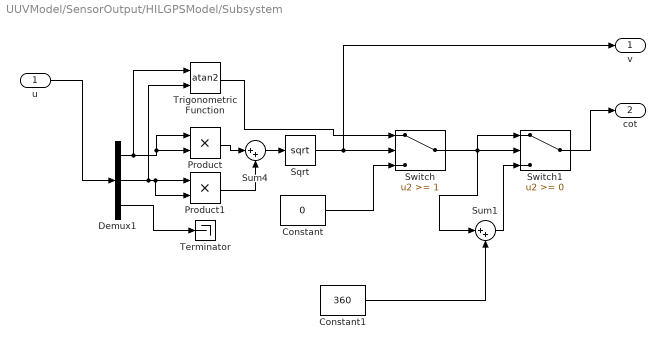
== system UUVModel/SensorOutput/HILGPSModel/Subsystem ==
  u : Inport
  Constant : Constant  Value=0
  Constant1 : Constant  Value=360
  Demux1 : Demux  Outputs=3
  Product : Product
  Product1 : Product
  Sqrt : Sqrt
  Sum1 : Sum  Inputs=|++
  Sum4 : Sum  Inputs=|++
  Switch : Switch  Threshold=1  SaturateOnIntegerOverflow=off  InputSameDT=off
  Switch1 : Switch  SaturateOnIntegerOverflow=off  InputSameDT=off
  Terminator : Terminator
  Trigonometric Function : Trigonometry  Operator=atan2
  v : Outport  VectorParamsAs1DForOutWhenUnconnected=off
  cot : Outport  Port=2  VectorParamsAs1DForOutWhenUnconnected=off
  wires:
  Demux1/2 -> Trigonometric Function/2, Product1/2, Product1/1
  Product/1 -> Sum4/1
  u/1 -> Demux1/1
  Switch/1 -> Sum1/1, Switch1/1, Switch1/2
  Product1/1 -> Sum4/2
  Demux1/3 -> Terminator/1
  Sqrt/1 -> v/1, Switch/2
  Constant/1 -> Switch/3
  Trigonometric Function/1 -> Switch/1
  Sum4/1 -> Sqrt/1
  Demux1/1 -> Trigonometric Function/1, Product/1, Product/2
  Constant1/1 -> Sum1/2
  Sum1/1 -> Switch1/3
  Switch1/1 -> cot/1

== system UUVModel/SensorOutput/HILSensorMavModel/GyroNoiseSwitch0 ==
  In1 : Inport
  Constant1 : Constant  Value=ModelParam_GlobalNoiseGainSwitch
  Constant2 : Constant  Value=0.2
  Gain2 : Gain  Gain=0.8
  Product4 : Product
  Sum : Sum  Inputs=|++
  Out1 : Outport  VectorParamsAs1DForOutWhenUnconnected=off
  wires:
  Sum/1 -> Product4/2
  Product4/1 -> Out1/1
  Gain2/1 -> Sum/1
  In1/1 -> Product4/1
  Constant1/1 -> Gain2/1
  Constant2/1 -> Sum/2

== system UUVModel/SensorOutput/HILSensorMavModel/GyroNoiseSwitch1 ==
  In1 : Inport
  Constant1 : Constant  Value=ModelParam_GlobalNoiseGainSwitch
  Constant2 : Constant  Value=0.2
  Gain2 : Gain  Gain=0.8
  Product4 : Product
  Sum : Sum  Inputs=|++
  Out1 : Outport  VectorParamsAs1DForOutWhenUnconnected=off
  wires:
  Sum/1 -> Product4/2
  Product4/1 -> Out1/1
  Gain2/1 -> Sum/1
  In1/1 -> Product4/1
  Constant1/1 -> Gain2/1
  Constant2/1 -> Sum/2

== system UUVModel/SensorOutput/HILSensorMavModel/GyroNoiseSwitch2 ==
  In1 : Inport
  Constant1 : Constant  Value=ModelParam_GlobalNoiseGainSwitch
  Constant2 : Constant  Value=0.2
  Gain2 : Gain  Gain=0.8
  Product4 : Product
  Sum : Sum  Inputs=|++
  Out1 : Outport  VectorParamsAs1DForOutWhenUnconnected=off
  wires:
  Sum/1 -> Product4/2
  Product4/1 -> Out1/1
  Gain2/1 -> Sum/1
  In1/1 -> Product4/1
  Constant1/1 -> Gain2/1
  Constant2/1 -> Sum/2

== system UUVModel/SensorOutput/HILSensorMavModel/GyroNoiseSwitch3 ==
  In1 : Inport
  Constant1 : Constant  Value=ModelParam_GlobalNoiseGainSwitch
  Constant2 : Constant  Value=0.3
  Gain2 : Gain  Gain=0.7
  Product4 : Product
  Sum : Sum  Inputs=|++
  Out1 : Outport  VectorParamsAs1DForOutWhenUnconnected=off
  wires:
  Sum/1 -> Product4/2
  Product4/1 -> Out1/1
  Gain2/1 -> Sum/1
  In1/1 -> Product4/1
  Constant1/1 -> Gain2/1
  Constant2/1 -> Sum/2

== system UUVModel/SensorOutput/HILSensorMavModel/GyroNoiseSwitch4 ==
  In1 : Inport
  Constant1 : Constant  Value=ModelParam_GlobalNoiseGainSwitch
  Constant2 : Constant  Value=0.3
  Gain2 : Gain  Gain=0.7
  Product4 : Product
  Sum : Sum  Inputs=|++
  Out1 : Outport  VectorParamsAs1DForOutWhenUnconnected=off
  wires:
  Sum/1 -> Product4/2
  Product4/1 -> Out1/1
  Gain2/1 -> Sum/1
  In1/1 -> Product4/1
  Constant1/1 -> Gain2/1
  Constant2/1 -> Sum/2

== matlab function UUVModel/Force and Moment Model/UUV/科里奥利（根据UUV） ==
  settings: updateMethod=DISCRETE
  data: Vb input; wb input; F3 output; M3 output; addedMassLinear input; addedMassAngular input
%{
function [F3,M3] = fcn(Vb,wb,...
    addedMassLinear,addedMassAngular)
% This is a ground model that can provides reaction force and reaction torque
% Vb=[1;-3.5;3];   % test
% wb=[0.5;0.6;-9.99];

%% 计算Coriolis力及力矩
Xudot = addedMassLinear(1);    % 对应参数addedMassLinear
Yvdot = addedMassLinear(2);
Zwdot = addedMassLinear(3);
Kpdot = addedMassAngular(1);    % 对应参数addedMassAngular
Mqdot = addedMassAngular(2);
Nrdot = addedMassAngular(3);
C_FA = [...
    0,Zwdot*Vb(3),-Yvdot*Vb(2);...
    -Zwdot*Vb(3),0,Xudot*Vb(1);...
    Yvdot*Vb(2),-Xudot*Vb(1),0];
C_TA = [...
    0,Nrdot*wb(3),-Mqdot*wb(2);...
    -Nrdot*wb(3),0,Kpdot*wb(1);...
    Mqdot*wb(2),-Kpdot*wb(1),0];

F3 = C_FA * wb;
M3 = C_FA * Vb + C_TA * wb;

% F3 = [0;0;0];
% M3 = [0;0;0];
% alpha = atan(Vb(3) / Vb(1));
% beta = asin(Vb(2) / sqrt(Vb(1)^2 + Vb(2)^2 + Vb(3)^2));
% v2 = dot(Vb,Vb);
% F3(1) = (K_D0 + K_D * alpha^2) * v2;
% F3(2) = K_beta * beta * v2;
% F3(3) = (K_L0 + K_L * alpha) * v2;
% M3(1) = (K_MY * beta + K_p * wb(1)) * v2;
% M3(2) = (K_M0 + K_M * alpha + K_q * wb(2)) * v2;
% M3(3) = (K_MZ * beta + K_r * wb(3)) * v2;

%}




function [F3, M3] = fcn(Vb, wb, addedMassLinear, addedMassAngular)
Vb = Vb(:); wb = wb(:);

% Diagonal terms (from inputs)
Xudot = addedMassLinear(1);
Yvdot = addedMassLinear(2);
Zwdot = addedMassLinear(3);
Kpdot = addedMassAngular(1);
Mqdot = addedMassAngular(2);
Nrdot = addedMassAngular(3);

% === 新增：典型交叉附加质量项（可标定）===
Yrdot = 0.6 * Yvdot;   % Y_{ṙ} ≈ 0.5~0.8 * Y_{v̇}
Zqdot = 0.6 * Zwdot;   % Z_{q̇} ≈ 0.5~0.8 * Z_{ẇ}
Nvdot = -0.8 * Nrdot;  % N_{v̇} ≈ -0.7~-1.0 * N_{ṙ}
Mwdot = -0.7 * Mqdot;  % M_{ẇ} ≈ -0.6~-0.9 * M_{q̇}
Xqdot = 0.2 * Xudot;   % X_{q̇} (small, due to pitch-induced surge)
Kwdot = 0.3 * Kpdot;   % K_{ẇ} (roll moment from heave)

% 构建完整的 6x6 附加质量矩阵 Ma
Ma = zeros(6);
% Diagonal
Ma(1,1) = Xudot;
Ma(2,2) = Yvdot;
Ma(3,3) = Zwdot;
Ma(4,4) = Kpdot;
Ma(5,5) = Mqdot;
Ma(6,6) = Nrdot;
% Off-diagonal (symmetric)
Ma(2,6) = Yrdot;   Ma(6,2) = Yrdot;   % Y_{ṙ} = N_{v̇} (reciprocal theorem)
Ma(3,5) = Zqdot;   Ma(5,3) = Zqdot;   % Z_{q̇} = M_{ẇ}
Ma(1,5) = Xqdot;   Ma(5,1) = Xqdot;   % X_{q̇} = M_{u̇}
Ma(3,4) = Kwdot;   Ma(4,3) = Kwdot;   % Z_{ṗ} = K_{ẇ}

% 广义速度
nu = [Vb; wb];

% 计算科里奥利矩阵 C_a (确保 skew-symmetric)
C_a = coriolis_from_Ma(Ma, nu);

% 总附加质量科里奥利力/力矩
tau_c = C_a * nu;
F3 = tau_c(1:3);
M3 = tau_c(4:6);
end

%% Helper: compute C_a from full Ma
function C = coriolis_from_Ma(Ma, nu)
v = nu(1:3); w = nu(4:6);
S_w = [0, -w(3), w(2); w(3), 0, -w(1); -w(2), w(1), 0];
S_v = [0, -v(3), v(2); v(3), 0, -v(1); -v(2), v(1), 0];
ad_nu = [S_w, zeros(3); S_v, S_w];
C = -ad_nu' * Ma - Ma * ad_nu + ad(Ma * nu)';
C = 0.5 * (C - C');  % enforce skew symmetry
end

function A = ad(xi)
v = xi(1:3); w = xi(4:6);
S_w = [0, -w(3), w(2); w(3), 0, -w(1); -w(2), w(1), 0];
S_v = [0, -v(3), v(2); v(3), 0, -v(1); -v(2), v(1), 0];
A = [S_w, zeros(3); S_v, S_w];
end

== matlab function UUVModel/Force and Moment Model/UUV/阻尼（根据UUV） ==
  settings: updateMethod=DISCRETE
  data: Vb input; wb input; F2 output; M2 output; dampingLinear input; dampingAngular input
%{
function [F2,M2] = fcn(Vb,wb,...
    dampingLinear,dampingAngular)
% This is a ground model that can provides reaction force and reaction torque
% Vb=[1;-3.5;3];   % test
% wb=[0.5;0.6;-9.99];
%% 计算阻尼
Xu = dampingLinear(1);    % 对应参数dampingLinear
Yv = dampingLinear(2);
Zw = dampingLinear(3);
Kp = dampingAngular(1);    % 对应参数dampingAngular
Mq = dampingAngular(2);
Nr = dampingAngular(3);

D_FL = [...
    -Xu,0,0;...
    0,-Yv,0;...
    0,0,-Zw];
D_FA = [...
    -Kp,0,0;...
    0,-Mq,0;...
    0,0,-Nr];

F2 = D_FL * Vb;
M2 = D_FA * wb;

% lambdas = [[ld11,ld12,ld13,ld14,ld15,ld16];[ld21,ld22,ld23,ld24,ld25,ld26];...
%            [ld31,ld32,ld33,ld34,ld35,ld36];[ld41,ld42,ld43,ld44,ld45,ld46];...
%            [ld51,ld52,ld53,ld54,ld55,ld56];[ld61,ld62,ld63,ld64,ld65,ld66]];
% temp = lambdas * [Vba;wba];
% F2 = temp(1:3);
% M2 = temp(4:6);
%}



function [F2, M2] = fcn(Vb, wb, dampingLinear, dampingAngular)
% High-fidelity damping model with:
% - Linear diagonal terms (from inputs)
% - Linear cross-coupling (built-in)
% - Quadratic (nonlinear) damping (hard-coded inside)
%
% Input interface unchanged: only 4 inputs!

% --- Enforce column vectors ---
Vb = Vb(:);
wb = wb(:);
dampingLinear = dampingLinear(:);
dampingAngular = dampingAngular(:);

% --- Validate input size ---
if length(Vb) ~= 3 || length(wb) ~= 3 || ...
   length(dampingLinear) ~= 3 || length(dampingAngular) ~= 3
    error('All inputs must be 3x1 vectors.');
end

% --- Assemble 6-DOF velocity ---
nu = [Vb; wb];  % [u; v; w; p; q; r]

% --- Build linear damping matrix D0 (6x6) with coupling ---
D0 = zeros(6);
D0(1,1) = dampingLinear(1);    % Xu
D0(2,2) = dampingLinear(2);    % Yv
D0(3,3) = dampingLinear(3);    % Zw
D0(4,4) = dampingAngular(1);   % Kp
D0(5,5) = dampingAngular(2);   % Mq
D0(6,6) = dampingAngular(3);   % Nr

% Hydrodynamic coupling (typical for slender AUVs)
D0(2,6) =  0.8 * dampingLinear(2);   % Y_r
D0(6,2) = -1.0 * dampingAngular(3);  % N_v
D0(3,5) =  0.6 * dampingLinear(3);   % Z_q
D0(5,3) = -0.8 * dampingAngular(2);  % M_w
D0(1,5) =  0.3 * dampingLinear(1);   % X_q
D0(5,1) = -0.4 * dampingAngular(2);  % M_u

% --- Hard-coded quadratic damping coefficients (6x1) ---
% Format: [Xu2; Yv2; Zw2; Kp2; Mq2; Nr2]
d_quad = [
    3.2;        % Xu2  (surge)
    7.5;        % Yv2  (sway)
    7.5;        % Zw2  (heave)
    0.0001;     % Kp2  (roll)
    0.001;      % Mq2  (pitch)
    0.001       % Nr2  (yaw)
];

% --- Compute nonlinear damping: d_i * |nu_i| * nu_i ---
nonlinear_damping = d_quad .* (abs(nu) .* nu);

% --- Total damping wrench ---
linear_damping = D0 * nu;
tau_d = -(linear_damping + nonlinear_damping);

% --- Outputs ---
F2 = tau_d(1:3);
M2 = tau_d(4:6);
end
